simulink model "sistema_furutaV2"  (R2024a)
settings: Solver=VariableStepAuto  StartTime=0.0  StopTime=2.5  RelTol=1e-3
values from neighbouring files (symbols this model uses):
  A = [A11 A12 A13 A14; A21 A22 A23 A24; A31 A32 A33 A34; A41 A42 A43 A44]    [FurutaLineal.m]    (also in ModeloFuruta.m = [0      0       1       0)
  B = [B11 B12; B21 B22; B31 B32; B41 B42]    [FurutaLineal.m]    (also in ModeloFuruta.m = [0)
  D = [2*I_x*block.ContStates.Data(4)*cos(block.ContStates.Data(2))*sin(block.ContStates.Data(2)), -C_z*M_2*l_bi*sin(block.ContStates.Data(2))*block.ContStates.Data(4); -I_x*block.ContStates.Data(3)*cos(block.ContStates.Data(2))*sin(block.ContStates.Data(2)), 0]    [FurutanolinealSLV2.m]
  K = 1.29    [FurutanolinealSLV2.m]
undefined symbols (not defined in the file or in its folder): A1, B1, C, C1, D1, K1
settings Model: Creator=PC  LastModifiedBy=juaco
settings SolverCC: MaxConsecutiveMinStep=100
settings RTWCC: GPUComputeCapability=3.5

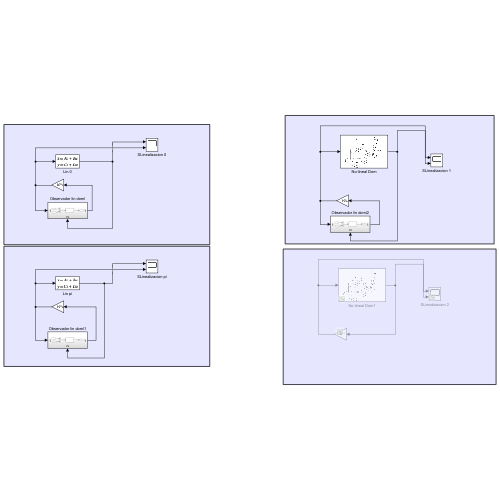
[thumbnail: Simulink's stored preview of the top-level diagram]
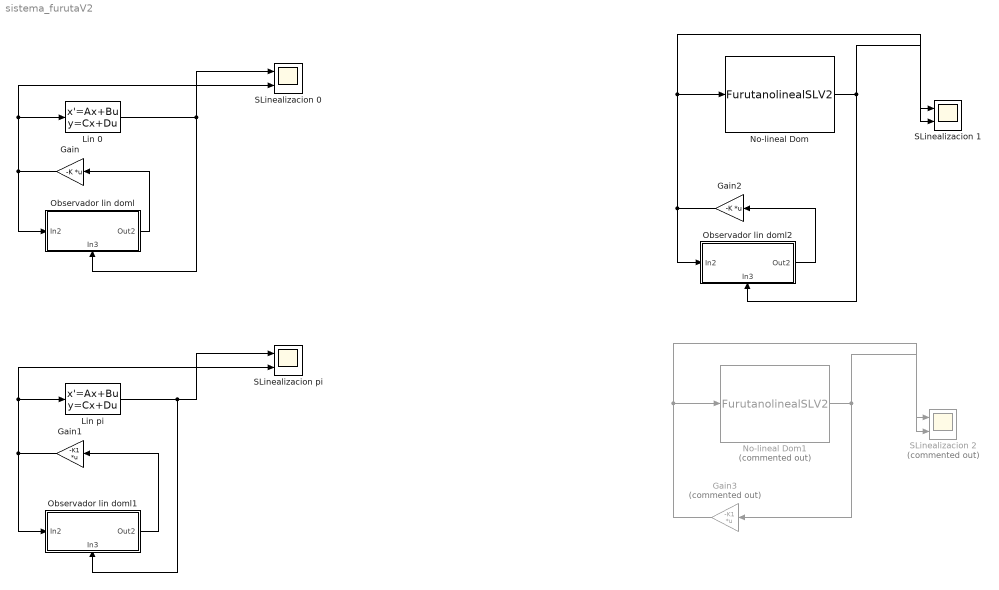
== system sistema_furutaV2 ==
  Gain : Gain  Gain=-K  Multiplication=Matrix(K*u)
  Gain1 : Gain  Gain=-K1  Multiplication=Matrix(K*u)
  Gain2 : Gain  Gain=-K  Multiplication=Matrix(K*u)
  Gain3 : Gain  Commented=on  Gain=-K1  Multiplication=Matrix(K*u)
  Lin 0 : StateSpace  A=A  B=B  C=C  D=D  InitialCondition=[0;0;0;0;0]  ParameterTunability=Unconstrained  AllowTunableDMatrix=on
  Lin pi : StateSpace  A=A1  B=B1  C=C1  D=D1  InitialCondition=[0;pi;0;0;0]  ParameterTunability=Unconstrained  AllowTunableDMatrix=on
  No-lineal Dom : M-S-Function  FunctionName=FurutanolinealSLV2  mask{Xi=0, g=0, J=0, M_2=0, l_bi=0, C_x=0, C_z=0, I_x=0, I_z=0}
      mask prompts: Xi "Parametros iniciales (Xi)"
      mask Display: image('mascara2.png');
  No-lineal Dom1 : M-S-Function  Commented=on  FunctionName=FurutanolinealSLV2  mask{Xi=0, g=0, J=0, M_2=0, l_bi=0, C_x=0, C_z=0, I_x=0, I_z=0}
      mask prompts: Xi "Parametros iniciales (Xi)"
      mask Display: image('mascara2.png');
  Observador lin doml : Subsystem
      settings: PortSchema="{\"entries\":[{\"content\":{\"sides\":[{\"content\":{\"connectorIds\":[\"In1\"]},\"type\":\"ConnectorPlacement.EquallySpacedRectSide\",\"uuid\":\"ba7a07d8-c095-4150-bb8b-07cf72cacb56\"},{\"content\":{\"connectorIds\":[\"Out1\"],\"side\":\"RIGHT\"},\"type\":\"ConnectorPlacement.EquallySpacedRectSide\",\"uuid\":\"0d1cce73-d5db-4a9e-9554-18b60846231f\"},{\"content\":{\"side\":\"TOP\"},\"type\":\"ConnectorPlacement.EquallySpacedRectSide\",\"uuid\":\"d3e5466d-f14f-4b11-b540-279949ac62cc\"},{\"content\":{\"connectorIds\":[\"In2\"],\"side\":\"BOTTOM\"},\"type\":\"ConnectorPlacement.EquallySpacedRectSide\",\"uuid\":\"b02fd88f-f8ea-43bc-a46b-088822b23831\"}]},\"type\":\"ConnectorPlacement.EquallySpacedConnector\",\"uuid\":\"b8204c46-8d4f-4ffa-96c5-dc8e990c325c\"}],\"packageUris\":[\"http://schema.mathworks.com/mf0/Connector/R2020b\"],\"version\":\"1.0\"}"
  Observador lin doml1 : Subsystem
      settings: PortSchema="{\"entries\":[{\"content\":{\"sides\":[{\"content\":{\"connectorIds\":[\"In1\"]},\"type\":\"ConnectorPlacement.EquallySpacedRectSide\",\"uuid\":\"ba7a07d8-c095-4150-bb8b-07cf72cacb56\"},{\"content\":{\"connectorIds\":[\"Out1\"],\"side\":\"RIGHT\"},\"type\":\"ConnectorPlacement.EquallySpacedRectSide\",\"uuid\":\"0d1cce73-d5db-4a9e-9554-18b60846231f\"},{\"content\":{\"side\":\"TOP\"},\"type\":\"ConnectorPlacement.EquallySpacedRectSide\",\"uuid\":\"d3e5466d-f14f-4b11-b540-279949ac62cc\"},{\"content\":{\"connectorIds\":[\"In2\"],\"side\":\"BOTTOM\"},\"type\":\"ConnectorPlacement.EquallySpacedRectSide\",\"uuid\":\"19f69271-4454-4d14-8b41-c9781e5bc8b7\"}]},\"type\":\"ConnectorPlacement.EquallySpacedConnector\",\"uuid\":\"b8204c46-8d4f-4ffa-96c5-dc8e990c325c\"}],\"packageUris\":[\"http://schema.mathworks.com/mf0/Connector/R2020b\"],\"version\":\"1.0\"}"
  Observador lin doml2 : Subsystem
      settings: PortSchema="{\"entries\":[{\"content\":{\"sides\":[{\"content\":{\"connectorIds\":[\"In1\"]},\"type\":\"ConnectorPlacement.EquallySpacedRectSide\",\"uuid\":\"ba7a07d8-c095-4150-bb8b-07cf72cacb56\"},{\"content\":{\"connectorIds\":[\"Out1\"],\"side\":\"RIGHT\"},\"type\":\"ConnectorPlacement.EquallySpacedRectSide\",\"uuid\":\"0d1cce73-d5db-4a9e-9554-18b60846231f\"},{\"content\":{\"side\":\"TOP\"},\"type\":\"ConnectorPlacement.EquallySpacedRectSide\",\"uuid\":\"d3e5466d-f14f-4b11-b540-279949ac62cc\"},{\"content\":{\"connectorIds\":[\"In2\"],\"side\":\"BOTTOM\"},\"type\":\"ConnectorPlacement.EquallySpacedRectSide\",\"uuid\":\"690de235-cc4b-4f83-9a56-1e06b3878d3c\"}]},\"type\":\"ConnectorPlacement.EquallySpacedConnector\",\"uuid\":\"b8204c46-8d4f-4ffa-96c5-dc8e990c325c\"}],\"packageUris\":[\"http://schema.mathworks.com/mf0/Connector/R2020b\"],\"version\":\"1.0\"}"
  SLinealizacion 0 : Scope  NumInputPorts=2
  SLinealizacion 1 : Scope  NumInputPorts=2
  SLinealizacion 2 : Scope  Commented=on  NumInputPorts=2
  SLinealizacion pi : Scope  NumInputPorts=2
  wires:
  Gain/1 -> Observador lin doml/1(In2), SLinealizacion 0/2, Lin 0/1
  Lin 0/1 -> SLinealizacion 0/1, Observador lin doml/2(In3)
  Lin pi/1 -> Observador lin doml1/2(In3), SLinealizacion pi/1
  Gain1/1 -> Observador lin doml1/1(In2), SLinealizacion pi/2, Lin pi/1
  No-lineal Dom/1 -> Observador lin doml2/2(In3), SLinealizacion 1/1
  Gain2/1 -> Observador lin doml2/1(In2), SLinealizacion 1/2, No-lineal Dom/1
  Gain3/1 -> SLinealizacion 2/2, No-lineal Dom1/1
  No-lineal Dom1/1 -> Gain3/1, SLinealizacion 2/1
  Observador lin doml1/1(Out2) -> Gain1/1
  Observador lin doml/1(Out2) -> Gain/1
  Observador lin doml2/1(Out2) -> Gain2/1

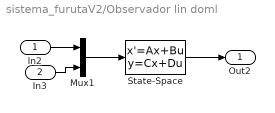
== system sistema_furutaV2/Observador lin doml ==
  In2 : Inport
  In3 : Inport  Port=2
  Mux1 : Mux  Inputs=2
  State-Space : StateSpace  A=[-40.5764905029500,-1.59337740152237,1.00000000000000,0,2.85954540723325;-1.62886658691906,-49.8671090961065,0,1.00000000000000,1.03580971180129;-7.56871003492383,-16.5915071451916,0,0,112.900732527960;-11.1524323314095,-229.815294972851,0,0,37.6091660270860;2.94244303428784,6.00953478090239,-15.3571428571429,0,-84.5564004009436]  B=[0,40.5764905029500,1.59337740152471,-2.85954540723325;0,1.62886658691906,49.8671090961797,-1.03580971180129;0,7.56871003492383,17.7189009854784,-72.6675743815088;0,11.1524323314095,327.135693657370,-3.22823691616955;11.9047619047619,-2.94244303428784,-6.00953478091121,-60.2055043609612]  C=[1,0,0,0,0;0,1,0,0,0;0,0,1,0,0;0,0,0,1,0;0,0,0,0,1]  D=[0,0,0,0;0,0,0,0;0,0,0,0;0,0,0,0;0,0,0,0]  InitialCondition=[0;pi;0;0;0]  ParameterTunability=Unconstrained  AllowTunableDMatrix=on
  Out2 : Outport
  wires:
  In2/1 -> Mux1/1
  State-Space/1 -> Out2/1
  Mux1/1 -> State-Space/1
  In3/1 -> Mux1/2

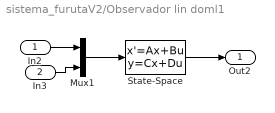
== system sistema_furutaV2/Observador lin doml1 ==
  In2 : Inport
  In3 : Inport  Port=2
  Mux1 : Mux  Inputs=2
  State-Space : StateSpace  A=[-40.5764905029500,-1.59337740152237,1.00000000000000,0,2.85954540723325;-1.62886658691906,-49.8671090961065,0,1.00000000000000,1.03580971180129;-7.56871003492383,-16.5915071451916,0,0,112.900732527960;-11.1524323314095,-229.815294972851,0,0,37.6091660270860;2.94244303428784,6.00953478090239,-15.3571428571429,0,-84.5564004009436]  B=[0,40.5764905029500,1.59337740152471,-2.85954540723325;0,1.62886658691906,49.8671090961797,-1.03580971180129;0,7.56871003492383,17.7189009854784,-72.6675743815088;0,11.1524323314095,327.135693657370,-3.22823691616955;11.9047619047619,-2.94244303428784,-6.00953478091121,-60.2055043609612]  C=[1,0,0,0,0;0,1,0,0,0;0,0,1,0,0;0,0,0,1,0;0,0,0,0,1]  D=[0,0,0,0;0,0,0,0;0,0,0,0;0,0,0,0;0,0,0,0]  InitialCondition=[0;pi;0;0;0]  ParameterTunability=Unconstrained  AllowTunableDMatrix=on
  Out2 : Outport
  wires:
  In2/1 -> Mux1/1
  State-Space/1 -> Out2/1
  Mux1/1 -> State-Space/1
  In3/1 -> Mux1/2

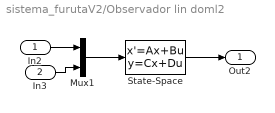
== system sistema_furutaV2/Observador lin doml2 ==
  In2 : Inport
  In3 : Inport  Port=2
  Mux1 : Mux  Inputs=2
  State-Space : StateSpace  A=[-40.5764905029500,-1.59337740152237,1.00000000000000,0,2.85954540723325;-1.62886658691906,-49.8671090961065,0,1.00000000000000,1.03580971180129;-7.56871003492383,-16.5915071451916,0,0,112.900732527960;-11.1524323314095,-229.815294972851,0,0,37.6091660270860;2.94244303428784,6.00953478090239,-15.3571428571429,0,-84.5564004009436]  B=[0,40.5764905029500,1.59337740152471,-2.85954540723325;0,1.62886658691906,49.8671090961797,-1.03580971180129;0,7.56871003492383,17.7189009854784,-72.6675743815088;0,11.1524323314095,327.135693657370,-3.22823691616955;11.9047619047619,-2.94244303428784,-6.00953478091121,-60.2055043609612]  C=[1,0,0,0,0;0,1,0,0,0;0,0,1,0,0;0,0,0,1,0;0,0,0,0,1]  D=[0,0,0,0;0,0,0,0;0,0,0,0;0,0,0,0;0,0,0,0]  InitialCondition=[0;pi;0;0;0]  ParameterTunability=Unconstrained  AllowTunableDMatrix=on
  Out2 : Outport
  wires:
  In2/1 -> Mux1/1
  State-Space/1 -> Out2/1
  Mux1/1 -> State-Space/1
  In3/1 -> Mux1/2
